simulink model "FaltaMonoAT_FaseCG"  (Simulink 10.3)
settings: Solver=ode23tb  StartTime=0.0  StopTime=100  RelTol=1e-4
values from neighbouring files (symbols this model uses):
  Pref_pu = 0.02    [powerReference.m]    (also in powerReferenceDesenergization.m)
  tbeg = 34    [Main_generateSimulations.m]
  tend = tbeg + ramdomValue(temporaryFaultDuration(1),temporaryFaultDuration(2))    [Main_generateSimulations.m]
  trig = 1e3    (= 1000)    [Main_generateSimulations.m]
  Vf0 = LF.sm.Vf    [Main_generateSimulations.m]
  Vref = Vt0    (= 1)    [Main_generateSimulations.m]
  Vt0 = abs(LF.sm.Vt)    [Main_generateSimulations.m]
undefined symbols (not defined in the file or in its folder): D1, Delta
libraries: spsLoadFlowBusLib x3, spsThreePhaseParallelRLCLoadLib x2, spsGroundLib x2, spsThreePhaseSourceLib x1, spsThreePhaseFaultLib x1, spsExcitationSystemLib x1, spsGroundingTransformerLib x1, spsHydraulicTurbineandGovernorLib x1, spsCurrentMeasurementLib x1, spsThreePhaseVIMeasurementLib x1, spsSynchronousMachinepuStandardLib x1, spsThreePhaseBreakerLib x1
Description:
  | Copyright 2008-2009 The MathWorks(TM), Inc.
settings Model: Creator=patrice  LastModifiedBy=cieslak  ExtModeTrigMode=oneshot  ExtModeArmWhenConnect=off  ExtModeAutoUpdateStatusClock=off
settings DataIOCC: SignalLoggingName=sigsOut
settings OptimizationCC: BlockReduction=off  BooleanDataType=off  InitFltsAndDblsToZero=on  EfficientMapNaN2IntZero=off
settings DebuggingCC: CheckExecutionContextPreStartOutputMsg=on  SignalResolutionControl=TryResolveAllWithWarning  MultiTaskDSMMsg=warning  MultiTaskCondExecSysMsg=none  SigSpecEnsureSampleTimeMsg=none
settings HardwareCC: TargetUnknown=on
settings SimscapeCC: SimscapeNormalizeSystem=off

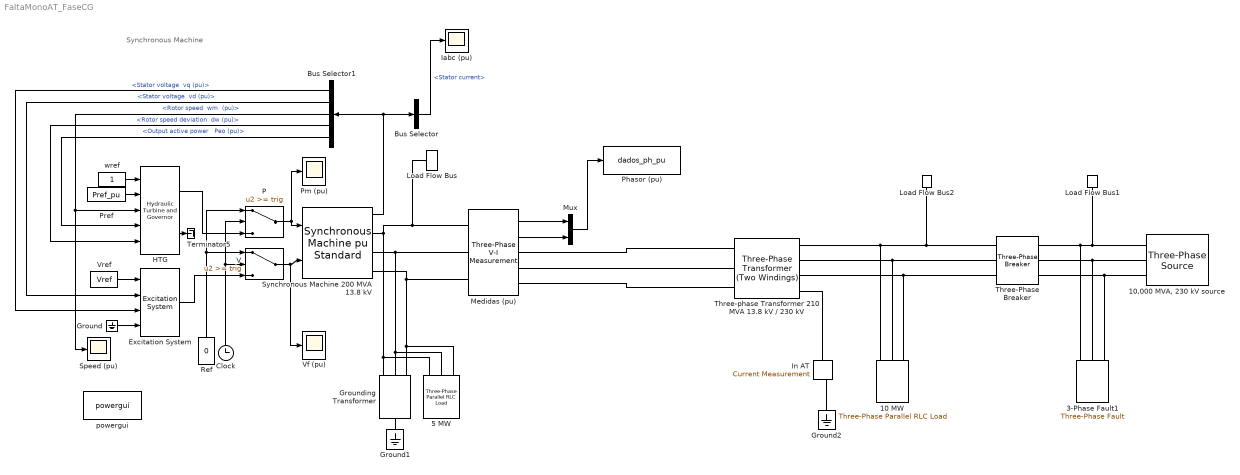
== system FaltaMonoAT_FaseCG ==
  note: Synchronous Machine
  " Iabc (pu)" : Scope
  " Speed (pu)" : Scope
  10 MW : spsThreePhaseParallelRLCLoadLib/Three-Phase Parallel RLC Load  LConnTagsString=A|B|C  Configuration=Y (grounded)  NominalVoltage=230e3  Vabc=[1e3 1e3 1e3]  Vabcp=[1e3 1e3 1e3]  NominalFrequency=60  UnbalancedPower=off  ActivePower=1e6  InductivePower=0  CapacitivePower=0  Pabc=[10e3 9e3 11e3]  QLabc=[100 90 110]  QCabc=[100 90 110]  Pabcp=[10e3 9e3 11e3]  QLabcp=[100 90 110]  QCabcp=[100 90 110]  Measurements=None  LoadType=constant Z
  "10,000 MVA, 230 kV source" : spsThreePhaseSourceLib/Three-Phase Source  InternalConnection=Yg  VoltagePhases=off  Voltage=230e3  PhaseAngle=0  Voltage_phases=[25e3 25e3 25e3]/sqrt(3)  PhaseAngles_phases=[0 -120 +120]  Frequency=60  NonIdealSource=on  SpecifyImpedance=on  Resistance=0.529  Inductance=0.0140  ShortCircuitLevel=10000e6  BaseVoltage=230e3  XRratio=10  BusType=swing  Pref=0  Qref=0  Prefabc=[10e3, 10e3, 10e3]  Qrefabc=[0, 0, 0]  Qmin=-inf  Qmax=inf
  3-Phase Fault1 : spsThreePhaseFaultLib/Three-Phase Fault  InitialStates=0  FaultA=off  FaultB=off  FaultC=on  GroundFault=on  SwitchTimes=[tbeg tend]  External=off  SwitchStatus=NaN  FaultResistance=Ron  GroundResistance=Rg  SnubberResistance=inf  SnubberCapacitance=inf  Measurements=None
  5 MW : spsThreePhaseParallelRLCLoadLib/Three-Phase Parallel RLC Load  LConnTagsString=A|B|C  Configuration=Y (grounded)  NominalVoltage=13.8e3  Vabc=[1e3 1e3 1e3]  Vabcp=[1e3 1e3 1e3]  NominalFrequency=60  UnbalancedPower=off  ActivePower=1e6  InductivePower=0  CapacitivePower=0  Pabc=[10e3 9e3 11e3]  QLabc=[100 90 110]  QCabc=[100 90 110]  Pabcp=[10e3 9e3 11e3]  QLabcp=[100 90 110]  QCabcp=[100 90 110]  Measurements=None  LoadType=constant Z
  Bus Selector : BusSelector  OutputSignals=Stator current
  Bus Selector1 : BusSelector  OutputSignals="dq0 components.Stator voltage  vq (pu),dq0 components.Stator voltage  vd (pu),Mechanical.Rotor speed  wm  (pu),Mechanical.Rotor speed deviation  dw (pu),Output active power   Peo (pu)"
  Clock : Clock
  Excitation System : spsExcitationSystemLib/Excitation System  tr=20e-3  reg=[ 300, 0.001 ]  exc=[ 1, 0 ]  tgr=[ 0, 0 ]  damp=[ 0.001, 0.1 ]  sat=[ 0, 0 ]  lim=[ -11.5, 11.5, 0 ]  v0=[Vt0 Vf0]
      settings: SourceProductBaseCode=PS
  Ground : Ground
  Ground1 : spsGroundLib/Ground  LConnTagsString=a
  Ground2 : spsGroundLib/Ground  LConnTagsString=a
  "Grounding Transformer " : spsGroundingTransformerLib/Grounding Transformer   UNITS=pu  NominalPower="[200e6   60]"  NominalVoltage=13.8e3  ZeroSequenceImpedance_pu=[0.025 0.075]  MagnetizationBranch_pu=[500 500]  ZeroSequenceImpedance_SI=[0.052083 589.05]  MagnetizationBranch_SI=[1041.7 3.927e+005]  Measurements=None
      settings: SourceProductBaseCode=PS
  HTG : spsHydraulicTurbineandGovernorLib/Hydraulic Turbine and Governor  sm="[ 10/3  0.07 ]"  gate="[  0.01  0.97518  -0.1  0.1 ]"  reg="[  0.05  1.163  0.105  0  0.01  ]"  hyd="[  0  2.67  ]"  dref=0  po=Pmec_pu
      settings: SourceProductBaseCode=PS
  In AT : spsCurrentMeasurementLib/Current Measurement  PhasorSimulation=on  OutputType=Complex  PSBequivalent=0
  Load Flow Bus : spsLoadFlowBusLib/Load Flow Bus  LConnTagsString=a  Phases=single  Connectors=on one side  ID=B1  Vbase=13.8e3  Vref=1  Vangle=0  VLF=1  VLFb=1  VLFc=1  angleLF=-23.07  angleLFb=0  angleLFc=0
      settings: SourceProductBaseCode=PS
  Load Flow Bus1 : spsLoadFlowBusLib/Load Flow Bus  LConnTagsString=a  Phases=single  Connectors=on one side  ID=B2  Vbase=230e3  Vref=1  Vangle=0  VLF=1  VLFb=1  VLFc=1  angleLF=0  angleLFb=0  angleLFc=0
      settings: AttributesFormatString=%<ID>\n%<Vbase>V\n%<VLF>pu\n%<angleLF>deg.  SourceProductBaseCode=PS
  Load Flow Bus2 : spsLoadFlowBusLib/Load Flow Bus  LConnTagsString=a  Phases=single  Connectors=on one side  ID=B3  Vbase=230e3  Vref=1  Vangle=0  VLF=1  VLFb=1  VLFc=1  angleLF=1.635e-05  angleLFb=0  angleLFc=0
      settings: AttributesFormatString=%<ID>\n%<Vbase>V\n%<VLF>pu\n%<angleLF>deg.  SourceProductBaseCode=PS
  Medidas (pu) : spsThreePhaseVIMeasurementLib/Three-Phase V-I Measurement  VoltageMeasurement=phase-to-ground  SetLabelV=off  LabelV=Vabc  Vpu=on  VpuLL=off  CurrentMeasurement=yes  SetLabelI=off  LabelI=Iabc  Ipu=on  Pbase=200e6  Vbase=13.8e3  OutputType=Complex  PhasorSimulation=on  PSBequivalent=0
  Mux : Mux  Inputs=2
  P : Switch  Threshold=trig
  Phasor (pu) : ToWorkspace  VariableName=dados_ph_pu  SaveFormat=Structure With Time  SampleTime=1/60
  Pm (pu) : Scope
  Pref : Constant  Value=Pref_pu
  Ref : Constant  Value=0
  Synchronous Machine 200 MVA 13.8 kV : spsSynchronousMachinepuStandardLib/Synchronous Machine pu Standard  PresetModel=No  MechanicalLoad=Mechanical power Pm  ShowDetailedParameters=on  RotorType=Salient-pole  Units=per unit standard parameters  MeasurementBus=off  NominalParameters="[ 200E6  13800   60 ]"  Reactances1=[ 31 32 33 34 35 36 37 ]  Reactances2=[ 1.305, 0.296, 0.252, 0.474, 0.243, 0.18 ]  dAxisTimeConstants=Short-circuit  qAxisTimeConstants=Open-circuit  TimeConstants1=[]  TimeConstants2=[]  TimeConstants3=[]  TimeConstants4=[]  TimeConstants5=[ 1.01, 0.053, 0.1 ]  TimeConstants6=[]  TimeConstants7=[]  TimeConstants8=[]  StatorResistance=2.8544e-3  Mechanical="[ 3.2 0  32]"  PolePairs=32  InitialConditions=[0 -93.5098 0.750193 0.750193 0.750193 -24.1939 -144.194 95.8061 1.29111]  SetSaturation=off  Saturation=[0.6404,0.7127,0.8441,0.9214,0.9956,1.082,1.19,1.316,1.457;0.7,0.7698,0.8872,0.9466,0.9969,1.046,1.1,1.151,1.201]  LoadFlowParameters=[1 150000000 0 0]  TsPowergui=0  TsBlock=-1  IterativeModel=Forward Euler  IterativeDiscreteModel=Trapezoidal non iterative  BusType=PQ  Pref=Pref  Qref=Qref  Qmin=-inf  Qmax=inf  PLF=0  QLF=0
      settings: SourceProductBaseCode=PS
  Terminator5 : Terminator
  Three-Phase Breaker : spsThreePhaseBreakerLib/Three-Phase Breaker  InitialState=closed  SwitchA=on  SwitchB=on  SwitchC=on  SwitchTimes=trig  External=off  BreakerResistance=0.001  SnubberResistance=1e6  SnubberCapacitance=inf  Measurements=None
  Three-phase Transformer 210 MVA 13.8 kV / 230 kV : spsThreePhaseTransformerTwoWindingsLib/Three-Phase Transformer (Two Windings)  Winding1Connection=Delta (D1)  Winding2Connection=Yn  CoreType=Three single-phase transformers  SetSaturation=off  Hysteresis=off  DataFile='hysteresis'  SetInitialFlux=off  Measurements=None  UNITS=pu  NominalPower=[ 210e6 60 ]  Winding1="[ 13.8e3 0.0027  0.08]"  Winding2=[ 230e3 0.0027 0.08]  Rm=500  Lm=500  L0=0.5  Saturation="[ 0,0  ;  0.005,1.2  ;  1.0,1.4 ]"  InitialFluxes=[ 0.8 , -0.8 , 0.7 ]  BreakLoop=off  DiscreteSolver=Trapezoidal iterative  DataType=off  TransfoNumber=0
  V : Switch  Threshold=trig
  Vf (pu) : Scope
  Vref : Constant  Value=Vref
  powergui : spspowerguiLib/powergui  Priority=2  SimulationMode=Phasor  SampleTime=0  frequency=60  Iterations=50  frequencyindice=60  Pbase=100e6  ErrMax=1e-4  UnitsV=kV  UnitsW=MW  buscounter=0  FunctionMessages=off  echomessages=off  EnableUseOfTLC=off  CurrentSourceSwitches=off  DisableSnubberDevices=off  DisableRonSwitches=off  DisableVfSwitches=off  DisplayEquations=off  AutomaticDiscreteSolvers=off  SolverType=Tustin  Interpol=off  ExternalGateDelay=off  methode=off  Ts=0  x0status=blocks  SPID=off  SwTol=0  HookPort=off  NonlinearTolerance=1e-4  nMaxIteration=100  ContinueOnMaxIteration=off  RestoreLinks=warning  ResistiveCurrentMeasurement=off  Frange=logspace(0,3,50)  Ylog=off  Xlog=off  ShowGrid=off  save=off  variable=ZData  structure=0  ZoomFFT=on  StartTime=0.0  cycles=2  DisplayStyle=off  fundamental=60  FreqAxis=off  MaxFrequency=1000  frequencyindicesteady=1  RmsSteady=1  display=off
  wref : Constant
  wires:
  Ground/1 -> Excitation System/4
  HTG/2 -> Terminator5/1
  Vref/1 -> Excitation System/1
  Pref/1 -> HTG/2
  wref/1 -> HTG/1
  Synchronous Machine 200 MVA 13.8 kV/1 -> Bus Selector/1, Bus Selector1/1
  Bus Selector/1 -> " Iabc (pu)"/1  "<Stator current>"
  Bus Selector1/1 -> Excitation System/3  "<Stator voltage  vq (pu)>"
  Bus Selector1/2 -> Excitation System/2  "<Stator voltage  vd (pu)>"
  Bus Selector1/3 -> HTG/3, " Speed (pu)"/1  "<Rotor speed  wm  (pu)>"
  Bus Selector1/4 -> HTG/5  "<Rotor speed deviation  dw (pu)>"
  Bus Selector1/5 -> HTG/4  "<Output active power   Peo (pu)>"
  P/1 -> Synchronous Machine 200 MVA 13.8 kV/1, Pm (pu)/1
  V/1 -> Vf (pu)/1, Synchronous Machine 200 MVA 13.8 kV/2
  HTG/1 -> P/3
  Excitation System/1 -> V/3
  Ref/1 -> V/1, P/1
  Clock/1 -> P/2, V/2
  Medidas (pu)/1 -> Mux/1
  Medidas (pu)/2 -> Mux/2
  Mux/1 -> Phasor (pu)/1
  connections:
  Medidas (pu)/LConn3 -- 5 MW/LConn3 -- "Grounding Transformer "/LConn3 -- Synchronous Machine 200 MVA 13.8 kV/RConn3
  "Grounding Transformer "/LConn2 -- 5 MW/LConn2 -- Medidas (pu)/LConn2 -- Synchronous Machine 200 MVA 13.8 kV/RConn2
  Synchronous Machine 200 MVA 13.8 kV/RConn1 -- Load Flow Bus/LConn1 -- Medidas (pu)/LConn1 -- 5 MW/LConn1 -- "Grounding Transformer "/LConn1
  Three-phase Transformer 210 MVA 13.8 kV / 230 kV/RConn3 -- 10 MW/LConn3 -- Three-Phase Breaker/LConn3
  Ground1/LConn1 -- "Grounding Transformer "/RConn1
  Three-phase Transformer 210 MVA 13.8 kV / 230 kV/RConn2 -- 10 MW/LConn2 -- Three-Phase Breaker/LConn2
  In AT/LConn1 -- Three-phase Transformer 210 MVA 13.8 kV / 230 kV/RConn4
  In AT/RConn1 -- Ground2/LConn1
  Three-Phase Breaker/RConn2 -- 3-Phase Fault1/LConn2 -- "10,000 MVA, 230 kV source"/RConn2
  "10,000 MVA, 230 kV source"/RConn1 -- Load Flow Bus1/LConn1 -- Three-Phase Breaker/RConn1 -- 3-Phase Fault1/LConn1
  "10,000 MVA, 230 kV source"/RConn3 -- 3-Phase Fault1/LConn3 -- Three-Phase Breaker/RConn3
  Three-phase Transformer 210 MVA 13.8 kV / 230 kV/LConn1 -- Medidas (pu)/RConn1
  Three-phase Transformer 210 MVA 13.8 kV / 230 kV/LConn2 -- Medidas (pu)/RConn2
  Three-phase Transformer 210 MVA 13.8 kV / 230 kV/LConn3 -- Medidas (pu)/RConn3
  Three-Phase Breaker/LConn1 -- Load Flow Bus2/LConn1 -- 10 MW/LConn1 -- Three-phase Transformer 210 MVA 13.8 kV / 230 kV/RConn1
